simulink model "accum_hdl_test"  (R2019b)
settings: Solver=FixedStepDiscrete  StartTime=0.0  StopTime=100  RelTol=1e-3
libraries: simulink x2, dspsrcs4 x1, lib_dsphdlcontrol_v1 x1
settings Model: DataTypeOverride=Off  Creator=mbabst  LastModifiedBy=mbabst
settings DataIOCC: SaveOutput=off  SaveTime=off  ReturnWorkspaceOutputs=off
settings OptimizationCC: BlockReduction=off  ConditionallyExecuteInputs=off  DefaultParameterBehavior=Inlined  LifeSpan=inf
settings DebuggingCC: AlgebraicLoopMsg=error  SingleTaskRateTransMsg=error  StrictBusMsg=ErrorOnBusTreatedAsVector  SFUnexpectedBacktrackingDiag=warning  SFNoUnconditionalDefaultTransitionDiag=warning  SFExecutionAtInitializationDiag=none  ArithmeticOperatorsInVariantConditions=warning
settings HardwareCC: ProdBitPerPointer=32  ProdBitPerSizeT=32  ProdBitPerPtrDiffT=32  ProdLargestAtomicFloat=None  ProdIntDivRoundTo=Undefined  ProdEndianess=Unspecified  ProdWordSize=32  ProdHWDeviceType=ASIC/FPGA->ASIC/FPGA  ProdEqTarget=off
settings SFSimCC: SimUseLocalCustomCode=off  CustomCodeUndefinedFunction=UseInterfaceOnly
settings RTWCC: RTWUseLocalCustomCode=off
settings CodeAppCC: StateflowObjectComments=on
settings GRTTargetCC: TargetLangStandard=C89/C90 (ANSI)
settings ConfigComp: CovMetricSettings=dw  CovHtmlReporting=on  CovSaveCumulativeToWorkspaceVar=on  CovSaveSingleToWorkspaceVar=on  CovExternalEMLEnable=off

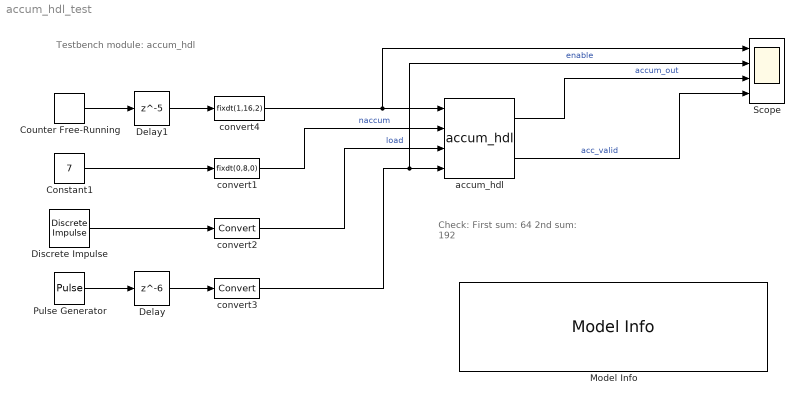
== system accum_hdl_test ==
  note: Testbench
      | module: accum_hdl
  note: Check:
      | First sum: 64
      | 2nd sum: 192
  Constant1 : Constant  Value=7  SampleTime=-1
  Counter Free-Running : simulink/Sources/Counter Free-Running  NumBits=16  tsamp=-1
  Delay : Delay  DelayLength=6  InitialCondition=0
  Delay1 : Delay  DelayLength=5  InitialCondition=0
  Discrete Impulse : dspsrcs4/Discrete  Impulse  Delay=2  SampleTime=1  FrameSample=1  OutputFrames=off  dataType=double  isSigned=on  wordLen=16  udDataType=sfix(16)  fracBitsMode=Best precision  numFracBits=15  OutDataTypeStr=double  LastOutDataTypeStr=double
  Model Info : simulink/Model-Wide Utilities/Model Info  Frame=on  DisplayStringWithTags=|  HorizontalTextAlignment=Left  LeftAlignmentValue=0.02
      | Copyright (c) 2005-2021 DSPlogic, Inc.
      | Distributed under the terms of the Simplified BSD License.
      | The full license is in the file LICENSE, distributed with this software.
      | 
      | Model: %<ModelName> (v%<ModelVersion>)
      | Author: Michael Babst <mike.babst@dsplogic.com>
      | Created: by %<Creator> on %<Created>
      | Modified: by %<ModifiedBy> on %<LastModificationDate>
  Pulse Generator : DiscretePulseGenerator
  Scope : Scope  NumInputPorts=4
  accum_hdl : lib_dsphdlcontrol_v1/accum_hdl  FreeRun=on
      settings: SourceProductName=DSPHDL Library
  convert1 : DataTypeConversion  OutDataTypeStr=fixdt(0,8,0)
  convert2 : DataTypeConversion
  convert3 : DataTypeConversion
  convert4 : DataTypeConversion  OutDataTypeStr=fixdt(1,16,2)  SaturateOnIntegerOverflow=on
  wires:
  Counter Free-Running/1 -> Delay1/1
  convert4/1 -> accum_hdl/1, Scope/1
  accum_hdl/1 -> Scope/3  "accum_out"
  Discrete Impulse/1 -> convert2/1
  Pulse Generator/1 -> Delay/1
  Constant1/1 -> convert1/1
  Delay/1 -> convert3/1
  convert1/1 -> accum_hdl/2  "naccum"
  convert2/1 -> accum_hdl/3  "load"
  convert3/1 -> accum_hdl/4, Scope/2  "enable"
  accum_hdl/2 -> Scope/4  "acc_valid"
  Delay1/1 -> convert4/1
